simulink model "LAB2_session5_PID"  (R2022b)
settings: Solver=VariableStepAuto  StartTime=0.0  StopTime=10.0  RelTol=1e-3
settings Model: Creator=Dell  LastModifiedBy=Dell

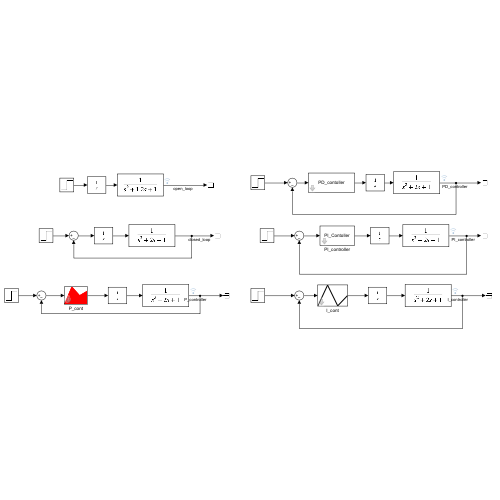
[thumbnail: Simulink's stored preview of the top-level diagram]
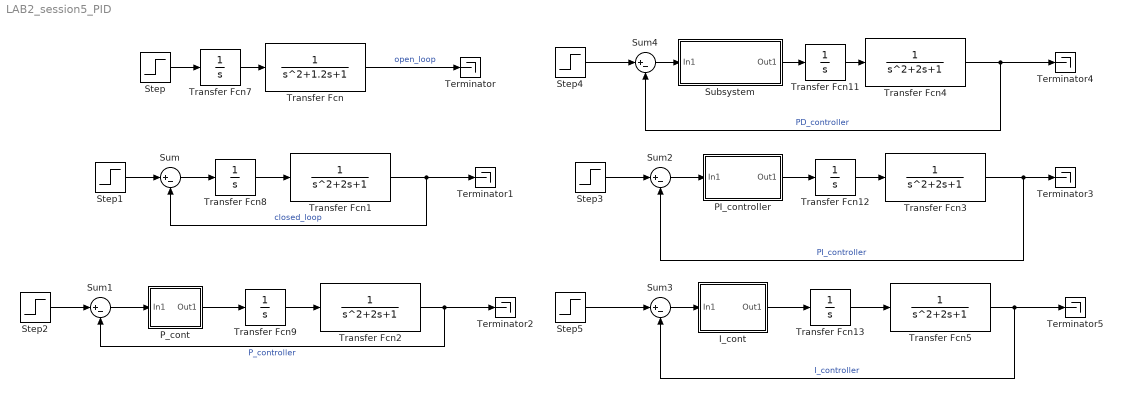
== system LAB2_session5_PID ==
  I_cont : Subsystem  mask{KI=0.5}
      mask Display:
      | plot([10 20 30 40], [10 20 10 15]);
      | color('red');
  PI_controller : Subsystem  mask{KP=1, KI=0.5}
      mask Display:
      | disp('PI_Contoller');
      | color('red');
  P_cont : Subsystem  mask{KP=1}
      mask Display:
      | patch([0 10 20 30 30 0], [10 30 20 25 10 10], [1 0 0]);
      | patch([0 10 20 30 30 0], [10 30 20 25 10 10], [1 0 0]);
  Step{,1..5} (6 alike) : Step  SampleTime=0
  Subsystem : Subsystem  mask{KP=0.5, KD=0.6}
      mask Display: disp('PD_contoller');
  Sum{,1..4} (5 alike) : Sum  Inputs=|+-
  Terminator{,1..5} (6 alike) : Terminator
  Transfer Fcn : TransferFcn  Denominator=[1 1.2 1]
  Transfer Fcn{1..5} (5 alike) : TransferFcn
  Transfer Fcn{7..9,11..13} (6 alike) : TransferFcn  Denominator=[1 0]
  wires:
  Transfer Fcn1/1 -> Sum/2, Terminator1/1  "closed_loop"
  Transfer Fcn4/1 -> Terminator4/1, Sum4/2  "PD_controller"
  Step4/1 -> Sum4/1
  Sum2/1 -> PI_controller/1(In1)
  Step2/1 -> Sum1/1
  Sum4/1 -> Subsystem/1(In1)
  Step/1 -> Transfer Fcn7/1
  Transfer Fcn5/1 -> Terminator5/1, Sum3/2  "I_controller"
  Transfer Fcn/1 -> Terminator/1  "open_loop"
  Transfer Fcn2/1 -> Sum1/2, Terminator2/1  "P_controller"
  PI_controller/1(Out1) -> Transfer Fcn12/1
  Transfer Fcn3/1 -> Sum2/2, Terminator3/1  "PI_controller"
  Sum3/1 -> I_cont/1(In1)
  Subsystem/1(Out1) -> Transfer Fcn11/1
  I_cont/1(Out1) -> Transfer Fcn13/1
  Step3/1 -> Sum2/1
  P_cont/1(Out1) -> Transfer Fcn9/1
  Step5/1 -> Sum3/1
  Sum1/1 -> P_cont/1(In1)
  Sum/1 -> Transfer Fcn8/1
  Step1/1 -> Sum/1
  Transfer Fcn7/1 -> Transfer Fcn/1
  Transfer Fcn8/1 -> Transfer Fcn1/1
  Transfer Fcn9/1 -> Transfer Fcn2/1
  Transfer Fcn11/1 -> Transfer Fcn4/1
  Transfer Fcn12/1 -> Transfer Fcn3/1
  Transfer Fcn13/1 -> Transfer Fcn5/1

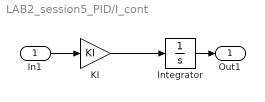
== system LAB2_session5_PID/I_cont ==
  In1 : Inport
  Integrator : Integrator
  KI : Gain  Gain=KI
  Out1 : Outport
  wires:
  KI/1 -> Integrator/1
  In1/1 -> KI/1
  Integrator/1 -> Out1/1

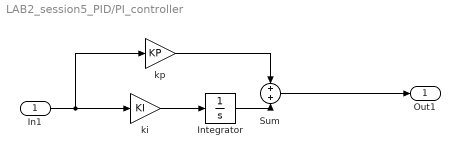
== system LAB2_session5_PID/PI_controller ==
  In1 : Inport
  Integrator : Integrator
  Sum : Sum
  ki : Gain  Gain=KI
  kp : Gain  Gain=KP
  Out1 : Outport
  wires:
  ki/1 -> Integrator/1
  kp/1 -> Sum/1
  Integrator/1 -> Sum/2
  Sum/1 -> Out1/1
  In1/1 -> kp/1, ki/1

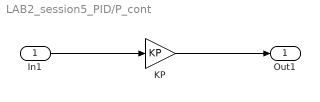
== system LAB2_session5_PID/P_cont ==
  In1 : Inport
  KP : Gain  Gain=KP
  Out1 : Outport
  wires:
  In1/1 -> KP/1
  KP/1 -> Out1/1

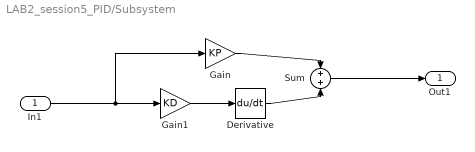
== system LAB2_session5_PID/Subsystem ==
  In1 : Inport
  Derivative : Derivative
  Gain : Gain  Gain=KP
  Gain1 : Gain  Gain=KD
  Sum : Sum
  Out1 : Outport
  wires:
  Gain1/1 -> Derivative/1
  Gain/1 -> Sum/1
  Derivative/1 -> Sum/2
  Sum/1 -> Out1/1
  In1/1 -> Gain/1, Gain1/1
